simulink library "idiada_lib"  (Simulink 8.1)
settings: Solver=ode1  StartTime=0.0  StopTime=Inf  FixedStep=0.001  RelTol=1e-3
PostLoadFcn:
  | , if any(exist('dsrtsu_mdlpostloadfcn', 'file') == [2, 3, 6]), try dsrtsu_mdlpostloadfcn('Execute', bdroot); catch fprintf('Error in PostLoadFcn (dsrtsu_mdlpostloadfcn) for model "%s":\n %s\n', bdroot, lasterr); end, end,
undefined symbols (not defined in the file or in its folder): C_TICK_TIME_S
settings Model: DSRTSU_INTERNAL_RTI_VER=450  DSRTSU_INTERNAL_RTI_TYPE=rti1401  RTICANMMDATA=struct('GeneralSetupData',struct('modelroot','D:\PROJECTS\HAITEC\TAIWAN_HAITEC_SVN\trunk\AdasDragon\software\sw_development\arch\util','generalsettings',struct('filesettings',struct('destfolder',struct('Name','RTICANMM_FILES','Check',1),'buildfolder',struct('Name','.','Check',1),'AbsDestfolder',struct('Name','D:\PROJECTS\HAITEC\TAIWAN_HAITEC_SVN\trunk\AdasDragon\software\sw_development\arch\util\RTICANMM_FILES'),'AbsBuildfolder',struct('Name','D:\PROJECTS\HAITEC\TAIWAN_HAITEC_SVN\trunk\AdasDragon\software\sw_development\arch\util'))),'options',struct('addpaths',1,'rmpaths',1,'addtrcexclusion',logical(1),'cannavigator',struct('checkmonitoring',0),'show_usrtrc',0,'use_usrtrc',0),'advanced',struct('options',[1 1 1 1 1 1 1 1 1 1 1 1 1 1 1 1 1 1 1 1 1 1 1 1 1 1 1 1 1 1 1 1 1 1 1 1 1 1 1 1 1 1 1 1 1 1 1 1 1 1 1 1 1 1 1 1 1 1 1 1 1 1 1 1 1 1 1 1 1 1 1 1 1 1 1 1 1 1 1 1 1 1 1 1 1 1 1 1 1 1 1 1 1 1 1 1 1 1 1 1]),'MPSetup',{{}},'modelname','idiada_lib','block','idiada_lib'))  DSRTSU_INTERNAL_RTIFPGA=40  Creator=AT015086  LastModifiedBy=tescamilla

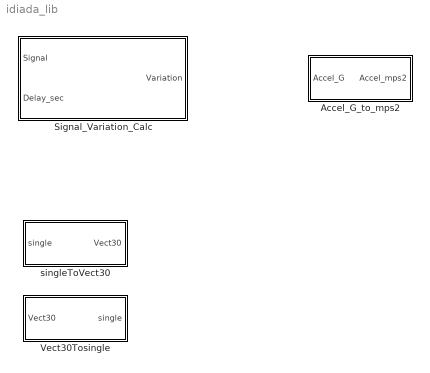
== system idiada_lib ==
  Accel_G_to_mps2 : Subsystem
  Signal_Variation_Calc : Subsystem
  Vect30Tosingle : Subsystem
  singleToVect30 : Subsystem

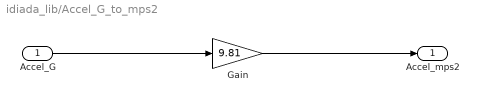
== system idiada_lib/Accel_G_to_mps2 ==
  Accel_G : Inport
  Gain : Gain  Gain=9.81
  Accel_mps2 : Outport
  wires:
  Accel_G/1 -> Gain/1
  Gain/1 -> Accel_mps2/1

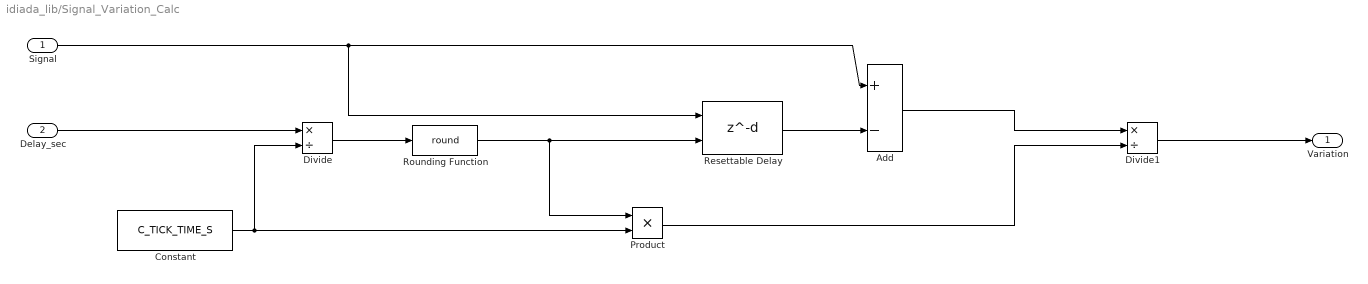
== system idiada_lib/Signal_Variation_Calc ==
  Signal : Inport
  Delay_sec : Inport  Port=2
  Add : Sum  Inputs=+-
  Constant : Constant  Value=C_TICK_TIME_S
  Divide : Product  Inputs=*/
  Divide1 : Product  Inputs=*/
  Product : Product
  Resettable Delay : Delay  DelayLengthSource=Input port  DelayLength=1  UseCircularBuffer=on
      settings: InputPortMap=u0,p1
  Rounding Function : Rounding  Operator=round
  Variation : Outport
  wires:
  Divide1/1 -> Variation/1
  Add/1 -> Divide1/1
  Delay_sec/1 -> Divide/1
  Rounding Function/1 -> Product/1, Resettable Delay/2
  Signal/1 -> Resettable Delay/1, Add/1
  Resettable Delay/1 -> Add/2
  Divide/1 -> Rounding Function/1
  Constant/1 -> Divide/2, Product/2
  Product/1 -> Divide1/2

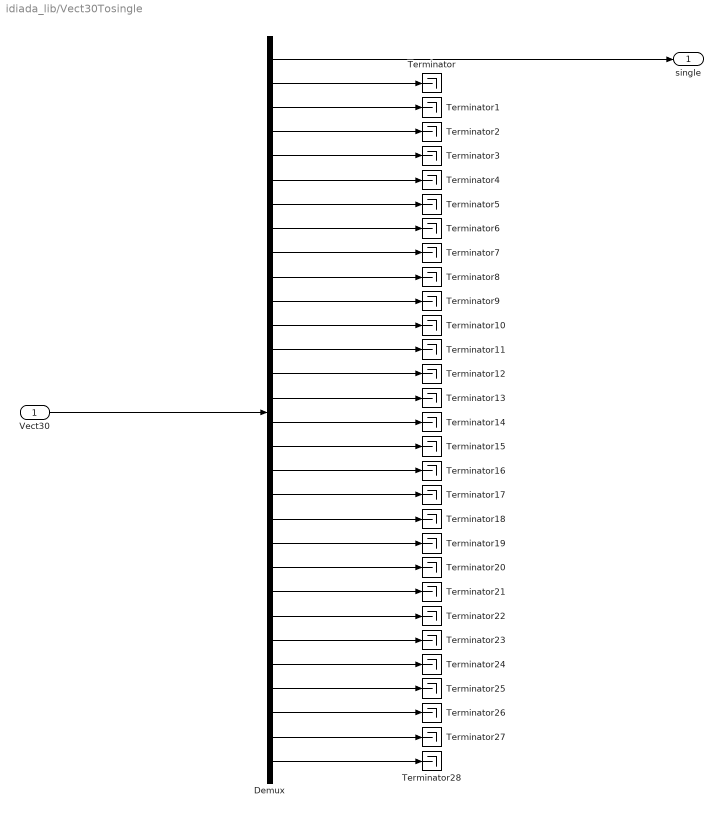
== system idiada_lib/Vect30Tosingle ==
  Vect30 : Inport
  Demux : Demux  Outputs=30
  Terminator{,1..28} (29 alike) : Terminator
  single : Outport
  wires:
  Demux/1 -> single/1
  Vect30/1 -> Demux/1
  Demux/2 -> Terminator/1
  Demux/3 -> Terminator1/1
  Demux/4 -> Terminator2/1
  Demux/5 -> Terminator3/1
  Demux/6 -> Terminator4/1
  Demux/7 -> Terminator5/1
  Demux/8 -> Terminator6/1
  Demux/9 -> Terminator7/1
  Demux/10 -> Terminator8/1
  Demux/11 -> Terminator9/1
  Demux/12 -> Terminator10/1
  Demux/13 -> Terminator11/1
  Demux/14 -> Terminator12/1
  Demux/15 -> Terminator13/1
  Demux/16 -> Terminator14/1
  Demux/17 -> Terminator15/1
  Demux/18 -> Terminator16/1
  Demux/19 -> Terminator17/1
  Demux/20 -> Terminator18/1
  Demux/21 -> Terminator19/1
  Demux/22 -> Terminator20/1
  Demux/23 -> Terminator21/1
  Demux/24 -> Terminator22/1
  Demux/25 -> Terminator23/1
  Demux/26 -> Terminator24/1
  Demux/27 -> Terminator25/1
  Demux/28 -> Terminator26/1
  Demux/29 -> Terminator27/1
  Demux/30 -> Terminator28/1

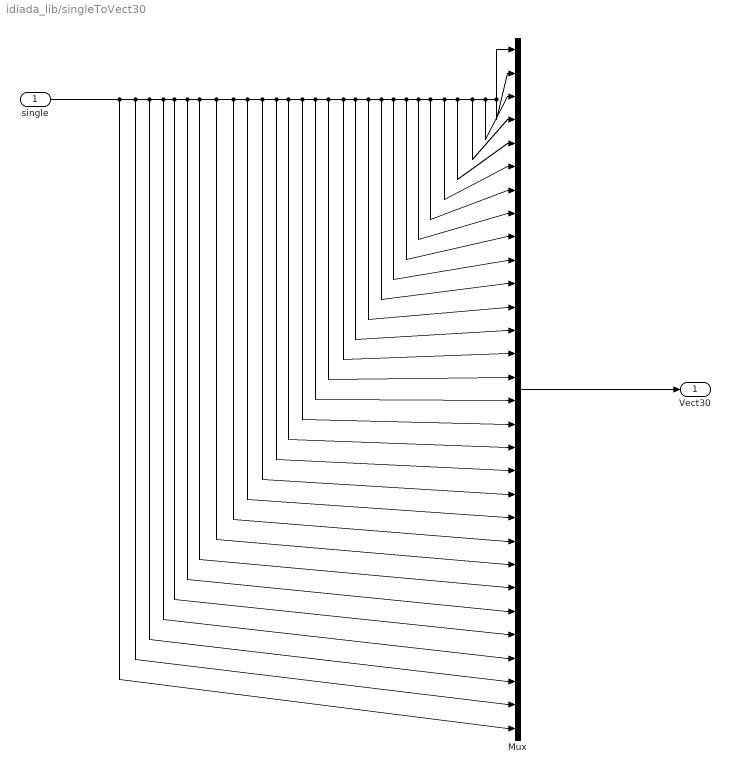
== system idiada_lib/singleToVect30 ==
  single : Inport
  Mux : Mux  Inputs=30
  Vect30 : Outport
  wires:
  single/1 -> Mux/30, Mux/29, Mux/28, Mux/1, Mux/2, Mux/3, Mux/4, Mux/5, Mux/6, Mux/7, Mux/8, Mux/9, Mux/10, Mux/11, Mux/12, Mux/13, Mux/14, Mux/15, Mux/16, Mux/17, Mux/18, Mux/19, Mux/20, Mux/21, Mux/22, Mux/23, Mux/24, Mux/25, Mux/26, Mux/27
  Mux/1 -> Vect30/1
